simulink model "laboratory3no2"  (R2023b)
settings: Solver=VariableStepAuto  StartTime=0.0  StopTime=10.0  RelTol=1e-3
settings Model: Creator=Emanuel  LastModifiedBy=Emanuel

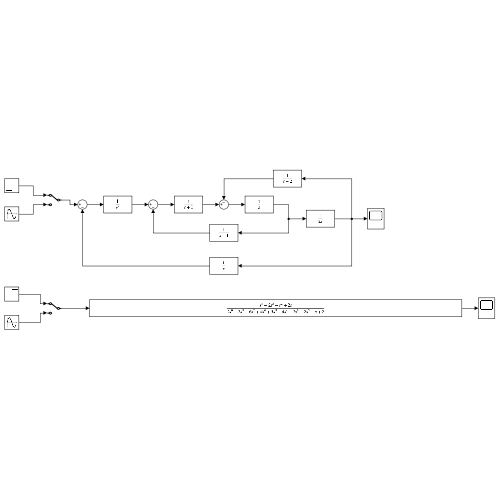
[thumbnail: Simulink's stored preview of the top-level diagram]
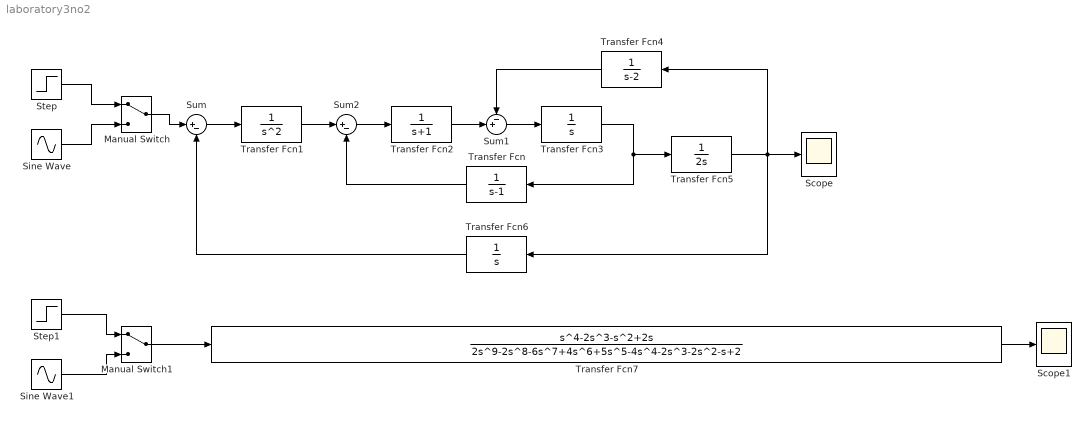
== system laboratory3no2 ==
  Manual Switch : ManualSwitch
  Manual Switch1 : ManualSwitch
  Scope : Scope
  Scope1 : Scope
  Sine Wave : Sin  SampleTime=0
  Sine Wave1 : Sin  SampleTime=0
  Step : Step  SampleTime=0
  Step1 : Step  SampleTime=0
  Sum : Sum  Inputs=|+-
  Sum1 : Sum  Inputs=-+|
  Sum2 : Sum  Inputs=|+-
  Transfer Fcn : TransferFcn  Denominator=[1 -1]
  Transfer Fcn1 : TransferFcn  Denominator=[1 0 0]
  Transfer Fcn2 : TransferFcn  Denominator=[1 1]
  Transfer Fcn3 : TransferFcn  Denominator=[1 0]
  Transfer Fcn4 : TransferFcn  Denominator=[1 -2]
  Transfer Fcn5 : TransferFcn  Denominator=[2 0]
  Transfer Fcn6 : TransferFcn  Denominator=[1 0]
  Transfer Fcn7 : TransferFcn  Numerator=[1 -2 -1 2 0]  Denominator=[2 -2 -6 4 5 -4 -2 -2 -1 2]
  wires:
  Sine Wave1/1 -> Manual Switch1/2
  Transfer Fcn7/1 -> Scope1/1
  Sum2/1 -> Transfer Fcn2/1
  Transfer Fcn5/1 -> Transfer Fcn6/1, Scope/1, Transfer Fcn4/1
  Transfer Fcn2/1 -> Sum1/2
  Sum/1 -> Transfer Fcn1/1
  Step/1 -> Manual Switch/1
  Transfer Fcn6/1 -> Sum/2
  Manual Switch/1 -> Sum/1
  Transfer Fcn1/1 -> Sum2/1
  Sum1/1 -> Transfer Fcn3/1
  Manual Switch1/1 -> Transfer Fcn7/1
  Transfer Fcn/1 -> Sum2/2
  Transfer Fcn4/1 -> Sum1/1
  Transfer Fcn3/1 -> Transfer Fcn/1, Transfer Fcn5/1
  Sine Wave/1 -> Manual Switch/2
  Step1/1 -> Manual Switch1/1
